simulink model "CIC_Filter_ISOP_HB"  (R2022b)
settings: Solver=FixedStepAuto  StartTime=0.0  StopTime=0.1  FixedStep=Ts/10  RelTol=1e-3
model workspace (MAT data in the model file):
  Ts = 1.953125e-06
  c = -6.248
  c6 = -5.494
settings Model: Creator=Rio  LastModifiedBy=Rio
settings DebuggingCC: ParameterPrecisionLossMsg=none

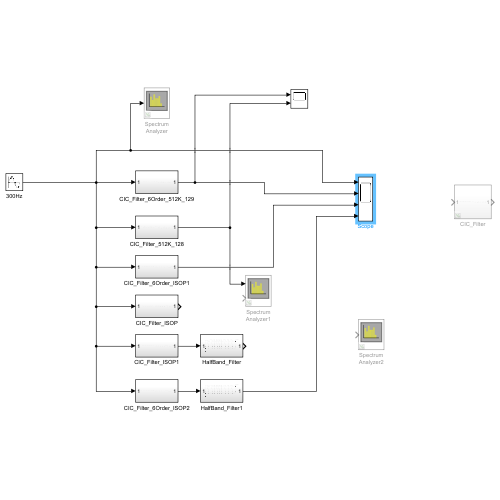
[thumbnail: Simulink's stored preview of the top-level diagram]
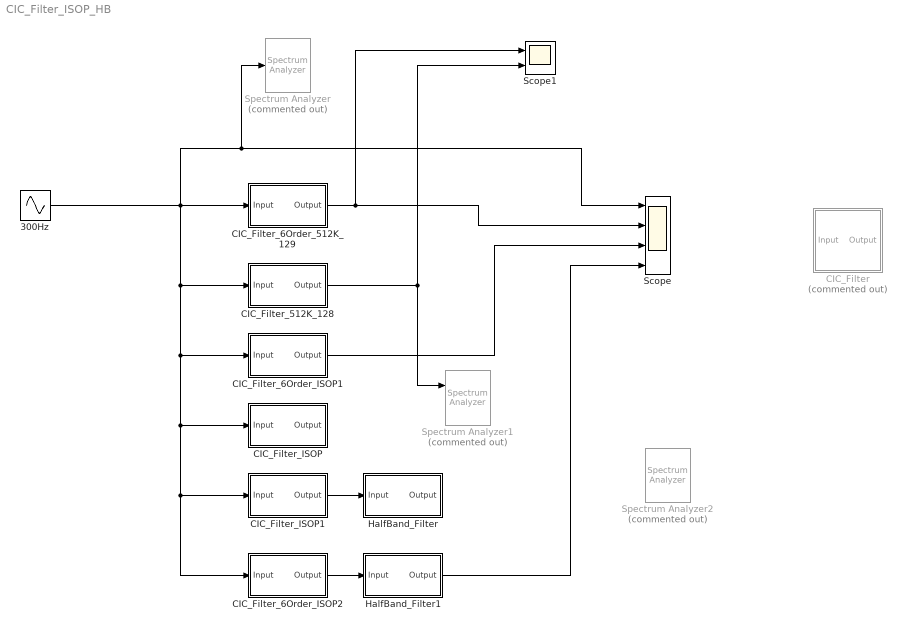
== system CIC_Filter_ISOP_HB ==
  300Hz : Sin  Frequency=2*pi*0  SampleTime=1/512000
  CIC_Filter : Subsystem  Commented=on
  CIC_Filter_512K_128 : Subsystem  Tag=FilterWizardSubSystem
      settings: ErrorFcn=dspFilterRealizedInBasicElemsAlgLoopErrFcnCallback
  CIC_Filter_6Order_512K_129 : Subsystem  Tag=FilterWizardSubSystem
      settings: ErrorFcn=dspFilterRealizedInBasicElemsAlgLoopErrFcnCallback
  CIC_Filter_6Order_ISOP1 : Subsystem  Tag=FilterWizardSubSystem
      settings: ErrorFcn=dspFilterRealizedInBasicElemsAlgLoopErrFcnCallback
  CIC_Filter_6Order_ISOP2 : Subsystem  Tag=FilterWizardSubSystem
      settings: ErrorFcn=dspFilterRealizedInBasicElemsAlgLoopErrFcnCallback
  CIC_Filter_ISOP : Subsystem  Tag=FilterWizardSubSystem
      settings: ErrorFcn=dspFilterRealizedInBasicElemsAlgLoopErrFcnCallback
  CIC_Filter_ISOP1 : Subsystem  Tag=FilterWizardSubSystem
      settings: ErrorFcn=dspFilterRealizedInBasicElemsAlgLoopErrFcnCallback
  HalfBand_Filter : Subsystem  Tag=FilterWizardSubSystem
      settings: ErrorFcn=dspFilterRealizedInBasicElemsAlgLoopErrFcnCallback
  HalfBand_Filter1 : Subsystem  Tag=FilterWizardSubSystem
      settings: ErrorFcn=dspFilterRealizedInBasicElemsAlgLoopErrFcnCallback
  Scope : Scope  NumInputPorts=4
  Scope1 : Scope  NumInputPorts=2
  Spectrum Analyzer : SpectrumAnalyzer  Commented=on
  Spectrum Analyzer1 : SpectrumAnalyzer  Commented=on  NumInputPorts=2
  Spectrum Analyzer2 : SpectrumAnalyzer  Commented=on
  wires:
  300Hz/1 -> CIC_Filter_6Order_512K_129/1(Input), CIC_Filter_6Order_ISOP1/1(Input), CIC_Filter_6Order_ISOP2/1(Input), CIC_Filter_ISOP1/1(Input), CIC_Filter_ISOP/1(Input), CIC_Filter_512K_128/1(Input), Scope/1, Spectrum Analyzer/1
  CIC_Filter_ISOP1/1(Output) -> HalfBand_Filter/1(Input)
  CIC_Filter_6Order_512K_129/1(Output) -> Scope1/1, Scope/2
  CIC_Filter_512K_128/1(Output) -> Spectrum Analyzer1/1, Scope1/2
  CIC_Filter_6Order_ISOP2/1(Output) -> HalfBand_Filter1/1(Input)
  CIC_Filter_6Order_ISOP1/1(Output) -> Scope/3
  HalfBand_Filter1/1(Output) -> Scope/4

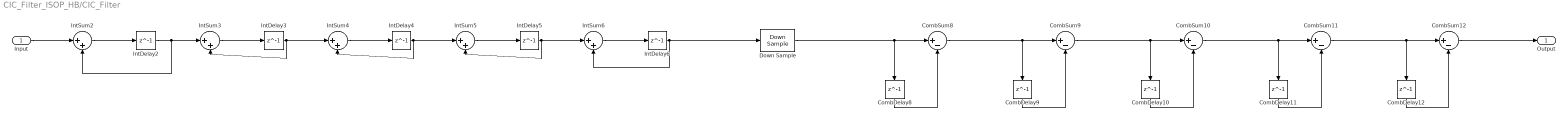
== system CIC_Filter_ISOP_HB/CIC_Filter ==
  Input : Inport
  CombDelay{8..12} (5 alike) : Delay  DelayLength=1  InitialCondition=0  SampleTime=Ts
  CombSum{8..12} (5 alike) : Sum  Inputs=|+-  AccumDataTypeStr=fixdt(1,51,15)  OutDataTypeStr=fixdt(1,51,15)
  Down Sample : DownSample  N=128  RateOptions=Allow multirate processing  AllowArbitraryFixedInput=on
  IntDelay{2..3,5..6} (4 alike) : Delay  DelayLength=1  InitialCondition=0  SampleTime=Ts
  IntDelay4 : Delay  DelayLength=1  InitialCondition=0
  IntSum{2..6} (5 alike) : Sum  Inputs=|++  AccumDataTypeStr=fixdt(1,51,15)  OutDataTypeStr=fixdt(1,51,15)
  Output : Outport
  wires:
  CombSum10/1 -> CombSum11/1, CombDelay11/1
  IntSum5/1 -> IntDelay5/1
  IntDelay4/1 -> IntSum4/2, IntSum5/1
  IntDelay6/1 -> IntSum6/2, Down Sample/1
  Down Sample/1 -> CombSum8/1, CombDelay8/1
  CombDelay12/1 -> CombSum12/2
  IntDelay5/1 -> IntSum5/2, IntSum6/1
  CombDelay8/1 -> CombSum8/2
  IntDelay3/1 -> IntSum3/2, IntSum4/1
  CombDelay11/1 -> CombSum11/2
  IntSum4/1 -> IntDelay4/1
  IntSum3/1 -> IntDelay3/1
  CombDelay10/1 -> CombSum10/2
  CombSum12/1 -> Output/1
  CombDelay9/1 -> CombSum9/2
  CombSum11/1 -> CombSum12/1, CombDelay12/1
  CombSum8/1 -> CombSum9/1, CombDelay9/1
  IntSum2/1 -> IntDelay2/1
  CombSum9/1 -> CombSum10/1, CombDelay10/1
  IntDelay2/1 -> IntSum2/2, IntSum3/1
  Input/1 -> IntSum2/1
  IntSum6/1 -> IntDelay6/1

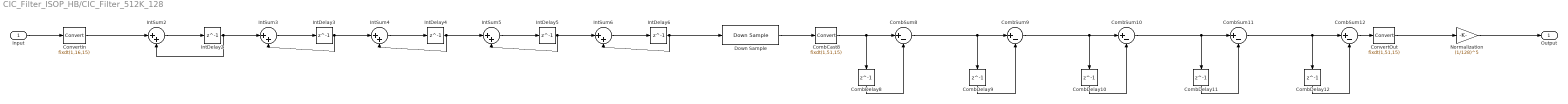
== system CIC_Filter_ISOP_HB/CIC_Filter_512K_128 ==
  Input : Inport
  CombCast8 : DataTypeConversion  OutDataTypeStr=fixdt(1,51,15)  SaturateOnIntegerOverflow=off  RndMeth=Floor
  CombDelay{8..12} (5 alike) : Delay  DelayLength=1  InitialCondition=0
  CombSum{8..12} (5 alike) : Sum  Inputs=|+-  AccumDataTypeStr=fixdt(1,51,15)  OutDataTypeStr=fixdt(1,51,15)
  ConvertIn : DataTypeConversion  OutDataTypeStr=fixdt(1,16,15)  RndMeth=Nearest
  ConvertOut : DataTypeConversion  OutDataTypeStr=fixdt(1,51,15)  SaturateOnIntegerOverflow=off  RndMeth=Floor
  Down Sample : DownSample  N=128  RateOptions=Allow multirate processing  AllowArbitraryFixedInput=on
  IntDelay{2..6} (5 alike) : Delay  DelayLength=1  InitialCondition=0
  IntSum{2..6} (5 alike) : Sum  Inputs=|++  AccumDataTypeStr=fixdt(1,51,15)  OutDataTypeStr=fixdt(1,51,15)
  Normalization : Gain  Gain=(1/128)^5
  Output : Outport
  wires:
  Input/1 -> ConvertIn/1
  IntSum2/1 -> IntDelay2/1
  IntDelay2/1 -> IntSum2/2, IntSum3/1
  IntSum3/1 -> IntDelay3/1
  IntDelay3/1 -> IntSum3/2, IntSum4/1
  IntSum4/1 -> IntDelay4/1
  IntDelay4/1 -> IntSum4/2, IntSum5/1
  IntSum5/1 -> IntDelay5/1
  IntDelay5/1 -> IntSum5/2, IntSum6/1
  IntSum6/1 -> IntDelay6/1
  IntDelay6/1 -> IntSum6/2, Down Sample/1
  Down Sample/1 -> CombCast8/1
  CombSum8/1 -> CombSum9/1, CombDelay9/1
  CombDelay8/1 -> CombSum8/2
  CombCast8/1 -> CombSum8/1, CombDelay8/1
  CombSum9/1 -> CombSum10/1, CombDelay10/1
  CombDelay9/1 -> CombSum9/2
  CombSum10/1 -> CombSum11/1, CombDelay11/1
  CombDelay10/1 -> CombSum10/2
  CombSum11/1 -> CombSum12/1, CombDelay12/1
  CombDelay11/1 -> CombSum11/2
  CombSum12/1 -> ConvertOut/1
  CombDelay12/1 -> CombSum12/2
  ConvertOut/1 -> Normalization/1
  ConvertIn/1 -> IntSum2/1
  Normalization/1 -> Output/1

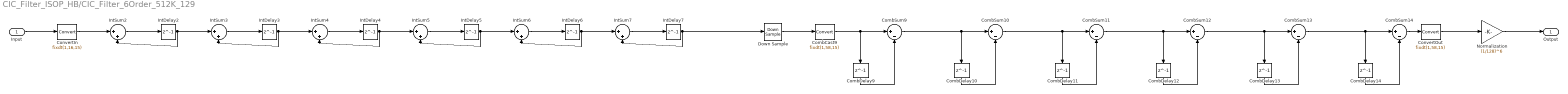
== system CIC_Filter_ISOP_HB/CIC_Filter_6Order_512K_129 ==
  Input : Inport
  CombCast9 : DataTypeConversion  OutDataTypeStr=fixdt(1,58,15)  SaturateOnIntegerOverflow=off  RndMeth=Floor
  CombDelay{9..14} (6 alike) : Delay  DelayLength=1  InitialCondition=0
  CombSum{9..14} (6 alike) : Sum  Inputs=|+-  AccumDataTypeStr=fixdt(1,58,15)  OutDataTypeStr=fixdt(1,58,15)
  ConvertIn : DataTypeConversion  OutDataTypeStr=fixdt(1,16,15)  RndMeth=Nearest
  ConvertOut : DataTypeConversion  OutDataTypeStr=fixdt(1,58,15)  SaturateOnIntegerOverflow=off  RndMeth=Floor
  Down Sample : DownSample  N=128  RateOptions=Allow multirate processing  AllowArbitraryFixedInput=on
  IntDelay{2..7} (6 alike) : Delay  DelayLength=1  InitialCondition=0
  IntSum{2..7} (6 alike) : Sum  Inputs=|++  AccumDataTypeStr=fixdt(1,58,15)  OutDataTypeStr=fixdt(1,58,15)
  Normalization : Gain  Gain=(1/128)^6
  Output : Outport
  wires:
  Input/1 -> ConvertIn/1
  ConvertIn/1 -> IntSum2/1
  IntSum2/1 -> IntDelay2/1
  IntDelay2/1 -> IntSum2/2, IntSum3/1
  IntSum3/1 -> IntDelay3/1
  IntDelay3/1 -> IntSum3/2, IntSum4/1
  IntSum4/1 -> IntDelay4/1
  IntDelay4/1 -> IntSum4/2, IntSum5/1
  IntSum5/1 -> IntDelay5/1
  IntDelay5/1 -> IntSum5/2, IntSum6/1
  IntSum6/1 -> IntDelay6/1
  IntDelay6/1 -> IntSum6/2, IntSum7/1
  IntSum7/1 -> IntDelay7/1
  IntDelay7/1 -> IntSum7/2, Down Sample/1
  Down Sample/1 -> CombCast9/1
  CombSum9/1 -> CombSum10/1, CombDelay10/1
  CombDelay9/1 -> CombSum9/2
  CombCast9/1 -> CombSum9/1, CombDelay9/1
  CombSum10/1 -> CombSum11/1, CombDelay11/1
  CombDelay10/1 -> CombSum10/2
  CombSum11/1 -> CombSum12/1, CombDelay12/1
  CombDelay11/1 -> CombSum11/2
  CombSum12/1 -> CombSum13/1, CombDelay13/1
  CombDelay12/1 -> CombSum12/2
  CombSum13/1 -> CombSum14/1, CombDelay14/1
  CombDelay13/1 -> CombSum13/2
  CombSum14/1 -> ConvertOut/1
  CombDelay14/1 -> CombSum14/2
  ConvertOut/1 -> Normalization/1
  Normalization/1 -> Output/1

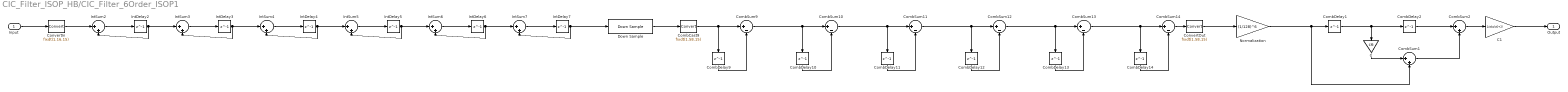
== system CIC_Filter_ISOP_HB/CIC_Filter_6Order_ISOP1 ==
  Input : Inport
  C : Gain  Gain=c6
  C1 : Gain  Gain=1/abs(c6+2)
  CombCast9 : DataTypeConversion  OutDataTypeStr=fixdt(1,58,15)  SaturateOnIntegerOverflow=off  RndMeth=Floor
  CombDelay{1..2,9..14} (8 alike) : Delay  DelayLength=1  InitialCondition=0
  CombSum1 : Sum  Inputs=|++  AccumDataTypeStr=fixdt(1,51,15)  OutDataTypeStr=fixdt(1,51,15)
  CombSum{9..14} (6 alike) : Sum  Inputs=|+-  AccumDataTypeStr=fixdt(1,58,15)  OutDataTypeStr=fixdt(1,58,15)
  CombSum2 : Sum  Inputs=|++  AccumDataTypeStr=fixdt(1,51,15)  OutDataTypeStr=fixdt(1,51,15)
  ConvertIn : DataTypeConversion  OutDataTypeStr=fixdt(1,16,15)  RndMeth=Nearest
  ConvertOut : DataTypeConversion  OutDataTypeStr=fixdt(1,58,15)  SaturateOnIntegerOverflow=off  RndMeth=Floor
  Down Sample : DownSample  N=128  RateOptions=Allow multirate processing  AllowArbitraryFixedInput=on
  IntDelay{2..7} (6 alike) : Delay  DelayLength=1  InitialCondition=0
  IntSum{2..7} (6 alike) : Sum  Inputs=|++  AccumDataTypeStr=fixdt(1,58,15)  OutDataTypeStr=fixdt(1,58,15)
  Normalization : Gain  Gain=(1/128)^6  OutDataTypeStr=Inherit: Same as input
  Output : Outport
  wires:
  ConvertOut/1 -> Normalization/1
  CombDelay14/1 -> CombSum14/2
  CombSum14/1 -> ConvertOut/1
  CombDelay13/1 -> CombSum13/2
  CombSum13/1 -> CombDelay14/1, CombSum14/1
  CombDelay12/1 -> CombSum12/2
  CombSum12/1 -> CombDelay13/1, CombSum13/1
  CombDelay11/1 -> CombSum11/2
  CombSum11/1 -> CombDelay12/1, CombSum12/1
  CombDelay10/1 -> CombSum10/2
  CombSum10/1 -> CombDelay11/1, CombSum11/1
  CombCast9/1 -> CombDelay9/1, CombSum9/1
  CombDelay9/1 -> CombSum9/2
  CombSum9/1 -> CombDelay10/1, CombSum10/1
  Down Sample/1 -> CombCast9/1
  IntDelay7/1 -> Down Sample/1, IntSum7/2
  IntSum7/1 -> IntDelay7/1
  IntDelay6/1 -> IntSum7/1, IntSum6/2
  IntSum6/1 -> IntDelay6/1
  IntDelay5/1 -> IntSum6/1, IntSum5/2
  IntSum5/1 -> IntDelay5/1
  IntDelay4/1 -> IntSum5/1, IntSum4/2
  IntSum4/1 -> IntDelay4/1
  IntDelay3/1 -> IntSum4/1, IntSum3/2
  IntSum3/1 -> IntDelay3/1
  IntDelay2/1 -> IntSum3/1, IntSum2/2
  IntSum2/1 -> IntDelay2/1
  ConvertIn/1 -> IntSum2/1
  Input/1 -> ConvertIn/1
  CombSum1/1 -> CombSum2/2
  CombDelay1/1 -> CombDelay2/1, C/1
  C1/1 -> Output/1
  C/1 -> CombSum1/1
  CombSum2/1 -> C1/1
  CombDelay2/1 -> CombSum2/1
  Normalization/1 -> CombDelay1/1, CombSum1/2

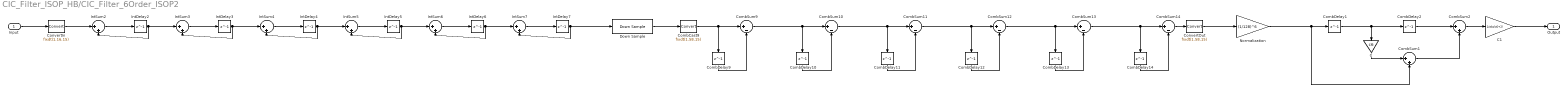
== system CIC_Filter_ISOP_HB/CIC_Filter_6Order_ISOP2 ==
  Input : Inport
  C : Gain  Gain=c6
  C1 : Gain  Gain=1/abs(c6+2)
  CombCast9 : DataTypeConversion  OutDataTypeStr=fixdt(1,58,15)  SaturateOnIntegerOverflow=off  RndMeth=Floor
  CombDelay{1..2,9..14} (8 alike) : Delay  DelayLength=1  InitialCondition=0
  CombSum1 : Sum  Inputs=|++  AccumDataTypeStr=fixdt(1,51,15)  OutDataTypeStr=fixdt(1,51,15)
  CombSum{9..14} (6 alike) : Sum  Inputs=|+-  AccumDataTypeStr=fixdt(1,58,15)  OutDataTypeStr=fixdt(1,58,15)
  CombSum2 : Sum  Inputs=|++  AccumDataTypeStr=fixdt(1,51,15)  OutDataTypeStr=fixdt(1,51,15)
  ConvertIn : DataTypeConversion  OutDataTypeStr=fixdt(1,16,15)  RndMeth=Nearest
  ConvertOut : DataTypeConversion  OutDataTypeStr=fixdt(1,58,15)  SaturateOnIntegerOverflow=off  RndMeth=Floor
  Down Sample : DownSample  N=128  RateOptions=Allow multirate processing  AllowArbitraryFixedInput=on
  IntDelay{2..7} (6 alike) : Delay  DelayLength=1  InitialCondition=0
  IntSum{2..7} (6 alike) : Sum  Inputs=|++  AccumDataTypeStr=fixdt(1,58,15)  OutDataTypeStr=fixdt(1,58,15)
  Normalization : Gain  Gain=(1/128)^6  OutDataTypeStr=Inherit: Same as input
  Output : Outport
  wires:
  Normalization/1 -> CombSum1/2, CombDelay1/1
  CombDelay2/1 -> CombSum2/1
  CombSum2/1 -> C1/1
  C/1 -> CombSum1/1
  C1/1 -> Output/1
  CombDelay1/1 -> C/1, CombDelay2/1
  CombSum1/1 -> CombSum2/2
  Input/1 -> ConvertIn/1
  ConvertIn/1 -> IntSum2/1
  IntSum2/1 -> IntDelay2/1
  IntDelay2/1 -> IntSum2/2, IntSum3/1
  IntSum3/1 -> IntDelay3/1
  IntDelay3/1 -> IntSum3/2, IntSum4/1
  IntSum4/1 -> IntDelay4/1
  IntDelay4/1 -> IntSum4/2, IntSum5/1
  IntSum5/1 -> IntDelay5/1
  IntDelay5/1 -> IntSum5/2, IntSum6/1
  IntSum6/1 -> IntDelay6/1
  IntDelay6/1 -> IntSum6/2, IntSum7/1
  IntSum7/1 -> IntDelay7/1
  IntDelay7/1 -> IntSum7/2, Down Sample/1
  Down Sample/1 -> CombCast9/1
  CombSum9/1 -> CombSum10/1, CombDelay10/1
  CombDelay9/1 -> CombSum9/2
  CombCast9/1 -> CombSum9/1, CombDelay9/1
  CombSum10/1 -> CombSum11/1, CombDelay11/1
  CombDelay10/1 -> CombSum10/2
  CombSum11/1 -> CombSum12/1, CombDelay12/1
  CombDelay11/1 -> CombSum11/2
  CombSum12/1 -> CombSum13/1, CombDelay13/1
  CombDelay12/1 -> CombSum12/2
  CombSum13/1 -> CombSum14/1, CombDelay14/1
  CombDelay13/1 -> CombSum13/2
  CombSum14/1 -> ConvertOut/1
  CombDelay14/1 -> CombSum14/2
  ConvertOut/1 -> Normalization/1

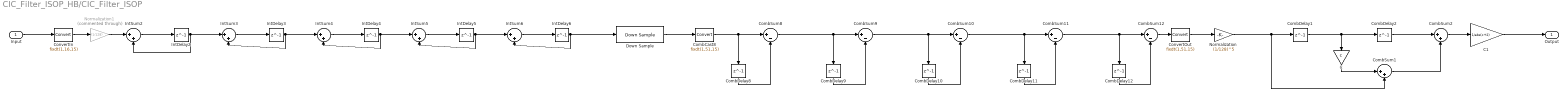
== system CIC_Filter_ISOP_HB/CIC_Filter_ISOP ==
  Input : Inport
  C : Gain  Gain=c
  C1 : Gain  Gain=1/abs(c+2)
  CombCast8 : DataTypeConversion  OutDataTypeStr=fixdt(1,51,15)  RndMeth=Floor
  CombDelay{1..2,8..12} (7 alike) : Delay  DelayLength=1  InitialCondition=0
  CombSum1 : Sum  Inputs=|++  AccumDataTypeStr=fixdt(1,51,15)  OutDataTypeStr=fixdt(1,51,15)
  CombSum{8..12} (5 alike) : Sum  Inputs=|+-  AccumDataTypeStr=fixdt(1,51,15)  OutDataTypeStr=fixdt(1,51,15)
  CombSum2 : Sum  Inputs=|++  AccumDataTypeStr=fixdt(1,51,15)  OutDataTypeStr=fixdt(1,51,15)
  ConvertIn : DataTypeConversion  OutDataTypeStr=fixdt(1,16,15)  RndMeth=Nearest
  ConvertOut : DataTypeConversion  OutDataTypeStr=fixdt(1,51,15)  RndMeth=Floor
  Down Sample : DownSample  N=128  RateOptions=Allow multirate processing  AllowArbitraryFixedInput=on
  IntDelay{2..6} (5 alike) : Delay  DelayLength=1  InitialCondition=0
  IntSum{2..6} (5 alike) : Sum  Inputs=|++  AccumDataTypeStr=fixdt(1,51,15)  OutDataTypeStr=fixdt(1,51,15)
  Normalization : Gain  Gain=(1/128)^5  OutDataTypeStr=Inherit: Same as input
  Normalization1 : Gain  Commented=through  Gain=(1/128)
  Output : Outport
  wires:
  Normalization/1 -> CombSum1/2, CombDelay1/1
  ConvertIn/1 -> Normalization1/1
  ConvertOut/1 -> Normalization/1
  CombDelay12/1 -> CombSum12/2
  CombSum12/1 -> ConvertOut/1
  CombDelay11/1 -> CombSum11/2
  CombSum11/1 -> CombDelay12/1, CombSum12/1
  CombDelay10/1 -> CombSum10/2
  CombSum10/1 -> CombDelay11/1, CombSum11/1
  CombDelay9/1 -> CombSum9/2
  CombSum9/1 -> CombDelay10/1, CombSum10/1
  CombCast8/1 -> CombDelay8/1, CombSum8/1
  CombDelay8/1 -> CombSum8/2
  CombSum8/1 -> CombDelay9/1, CombSum9/1
  Down Sample/1 -> CombCast8/1
  IntDelay6/1 -> Down Sample/1, IntSum6/2
  IntSum6/1 -> IntDelay6/1
  IntDelay5/1 -> IntSum6/1, IntSum5/2
  IntSum5/1 -> IntDelay5/1
  IntDelay4/1 -> IntSum5/1, IntSum4/2
  IntSum4/1 -> IntDelay4/1
  IntDelay3/1 -> IntSum4/1, IntSum3/2
  IntSum3/1 -> IntDelay3/1
  IntDelay2/1 -> IntSum3/1, IntSum2/2
  IntSum2/1 -> IntDelay2/1
  Input/1 -> ConvertIn/1
  CombDelay1/1 -> CombDelay2/1, C/1
  C/1 -> CombSum1/1
  CombSum1/1 -> CombSum2/2
  CombDelay2/1 -> CombSum2/1
  CombSum2/1 -> C1/1
  Normalization1/1 -> IntSum2/1
  C1/1 -> Output/1

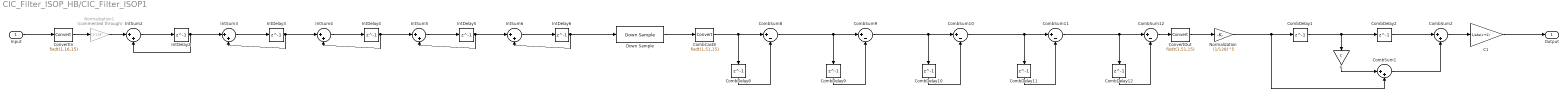
== system CIC_Filter_ISOP_HB/CIC_Filter_ISOP1 ==
  Input : Inport
  C : Gain  Gain=c
  C1 : Gain  Gain=1/abs(c+2)
  CombCast8 : DataTypeConversion  OutDataTypeStr=fixdt(1,51,15)  RndMeth=Floor
  CombDelay{1..2,8..12} (7 alike) : Delay  DelayLength=1  InitialCondition=0
  CombSum1 : Sum  Inputs=|++  AccumDataTypeStr=fixdt(1,51,15)  OutDataTypeStr=fixdt(1,51,15)
  CombSum{8..12} (5 alike) : Sum  Inputs=|+-  AccumDataTypeStr=fixdt(1,51,15)  OutDataTypeStr=fixdt(1,51,15)
  CombSum2 : Sum  Inputs=|++  AccumDataTypeStr=fixdt(1,51,15)  OutDataTypeStr=fixdt(1,51,15)
  ConvertIn : DataTypeConversion  OutDataTypeStr=fixdt(1,16,15)  RndMeth=Nearest
  ConvertOut : DataTypeConversion  OutDataTypeStr=fixdt(1,51,15)  RndMeth=Floor
  Down Sample : DownSample  N=128  RateOptions=Allow multirate processing  AllowArbitraryFixedInput=on
  IntDelay{2..6} (5 alike) : Delay  DelayLength=1  InitialCondition=0
  IntSum{2..6} (5 alike) : Sum  Inputs=|++  AccumDataTypeStr=fixdt(1,51,15)  OutDataTypeStr=fixdt(1,51,15)
  Normalization : Gain  Gain=(1/128)^5  OutDataTypeStr=Inherit: Same as input
  Normalization1 : Gain  Commented=through  Gain=(1/128)
  Output : Outport
  wires:
  C1/1 -> Output/1
  Normalization1/1 -> IntSum2/1
  CombSum2/1 -> C1/1
  CombDelay2/1 -> CombSum2/1
  CombSum1/1 -> CombSum2/2
  C/1 -> CombSum1/1
  CombDelay1/1 -> C/1, CombDelay2/1
  Input/1 -> ConvertIn/1
  IntSum2/1 -> IntDelay2/1
  IntDelay2/1 -> IntSum2/2, IntSum3/1
  IntSum3/1 -> IntDelay3/1
  IntDelay3/1 -> IntSum3/2, IntSum4/1
  IntSum4/1 -> IntDelay4/1
  IntDelay4/1 -> IntSum4/2, IntSum5/1
  IntSum5/1 -> IntDelay5/1
  IntDelay5/1 -> IntSum5/2, IntSum6/1
  IntSum6/1 -> IntDelay6/1
  IntDelay6/1 -> IntSum6/2, Down Sample/1
  Down Sample/1 -> CombCast8/1
  CombSum8/1 -> CombSum9/1, CombDelay9/1
  CombDelay8/1 -> CombSum8/2
  CombCast8/1 -> CombSum8/1, CombDelay8/1
  CombSum9/1 -> CombSum10/1, CombDelay10/1
  CombDelay9/1 -> CombSum9/2
  CombSum10/1 -> CombSum11/1, CombDelay11/1
  CombDelay10/1 -> CombSum10/2
  CombSum11/1 -> CombSum12/1, CombDelay12/1
  CombDelay11/1 -> CombSum11/2
  CombSum12/1 -> ConvertOut/1
  CombDelay12/1 -> CombSum12/2
  ConvertOut/1 -> Normalization/1
  ConvertIn/1 -> Normalization1/1
  Normalization/1 -> CombDelay1/1, CombSum1/2

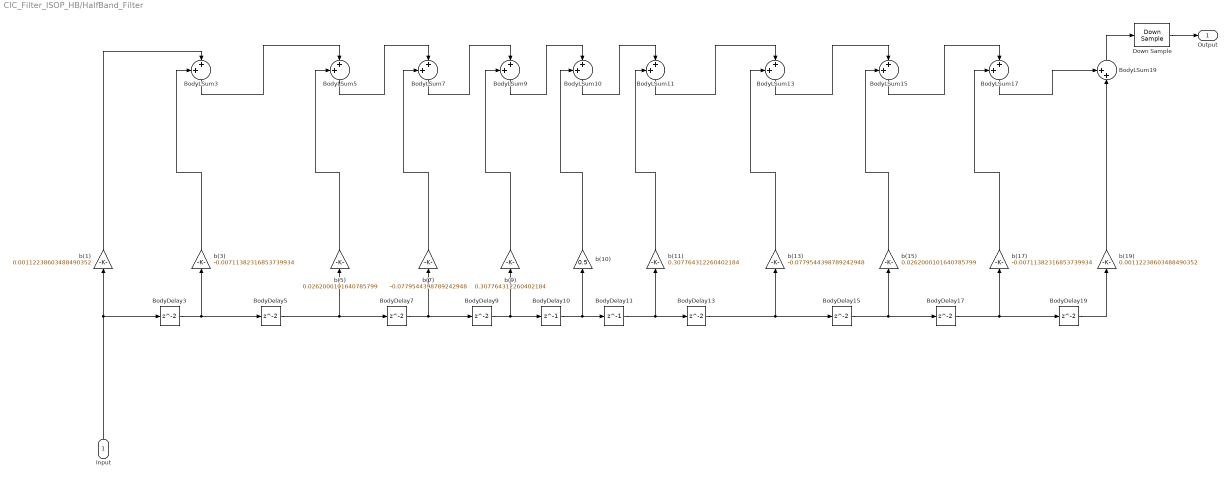
== system CIC_Filter_ISOP_HB/HalfBand_Filter ==
  Input : Inport
  BodyDelay10 : Delay  DelayLength=1  InitialCondition=0  InputProcessing=Columns as channels (frame based)
  BodyDelay11 : Delay  DelayLength=1  InitialCondition=0  InputProcessing=Columns as channels (frame based)
  BodyDelay{3,5,7,9,13,15,17,19} (8 alike) : Delay  InitialCondition=0  InputProcessing=Columns as channels (frame based)
  BodyLSum{3,5,7,9..11,13,15,17,19} (10 alike) : Sum  Inputs=++|  RndMeth=Nearest  SaturateOnIntegerOverflow=on  OutDataTypeStr=Inherit: Same as first input
  Down Sample : DownSample  RateOptions=Allow multirate processing  AllowArbitraryFixedInput=on
  b(1) : Gain  Gain=0.00112238603488490352  ParamDataTypeStr=single  RndMeth=Nearest  SaturateOnIntegerOverflow=on  OutDataTypeStr=Inherit: Same as input
  b(10) : Gain  Gain=0.5  ParamDataTypeStr=single  RndMeth=Nearest  SaturateOnIntegerOverflow=on  OutDataTypeStr=Inherit: Same as input
  b(11) : Gain  Gain=0.307764312260402184  ParamDataTypeStr=single  RndMeth=Nearest  SaturateOnIntegerOverflow=on  OutDataTypeStr=Inherit: Same as input
  b(13) : Gain  Gain=-0.0779544398789242948  ParamDataTypeStr=single  RndMeth=Nearest  SaturateOnIntegerOverflow=on  OutDataTypeStr=Inherit: Same as input
  b(15) : Gain  Gain=0.0262000101640785799  ParamDataTypeStr=single  RndMeth=Nearest  SaturateOnIntegerOverflow=on  OutDataTypeStr=Inherit: Same as input
  b(17) : Gain  Gain=-0.00711382316853739934  ParamDataTypeStr=single  RndMeth=Nearest  SaturateOnIntegerOverflow=on  OutDataTypeStr=Inherit: Same as input
  b(19) : Gain  Gain=0.00112238603488490352  ParamDataTypeStr=single  RndMeth=Nearest  SaturateOnIntegerOverflow=on  OutDataTypeStr=Inherit: Same as input
  b(3) : Gain  Gain=-0.00711382316853739934  ParamDataTypeStr=single  RndMeth=Nearest  SaturateOnIntegerOverflow=on  OutDataTypeStr=Inherit: Same as input
  b(5) : Gain  Gain=0.0262000101640785799  ParamDataTypeStr=single  RndMeth=Nearest  SaturateOnIntegerOverflow=on  OutDataTypeStr=Inherit: Same as input
  b(7) : Gain  Gain=-0.0779544398789242948  ParamDataTypeStr=single  RndMeth=Nearest  SaturateOnIntegerOverflow=on  OutDataTypeStr=Inherit: Same as input
  b(9) : Gain  Gain=0.307764312260402184  ParamDataTypeStr=single  RndMeth=Nearest  SaturateOnIntegerOverflow=on  OutDataTypeStr=Inherit: Same as input
  Output : Outport
  wires:
  Input/1 -> b(1)/1, BodyDelay3/1
  b(1)/1 -> BodyLSum3/2
  BodyDelay3/1 -> b(3)/1, BodyDelay5/1
  b(3)/1 -> BodyLSum3/1
  BodyLSum3/1 -> BodyLSum5/2
  BodyDelay5/1 -> b(5)/1, BodyDelay7/1
  b(5)/1 -> BodyLSum5/1
  BodyLSum5/1 -> BodyLSum7/2
  BodyDelay7/1 -> b(7)/1, BodyDelay9/1
  b(7)/1 -> BodyLSum7/1
  BodyLSum7/1 -> BodyLSum9/2
  BodyDelay9/1 -> b(9)/1, BodyDelay10/1
  b(9)/1 -> BodyLSum9/1
  BodyLSum9/1 -> BodyLSum10/2
  BodyDelay10/1 -> b(10)/1, BodyDelay11/1
  b(10)/1 -> BodyLSum10/1
  BodyLSum10/1 -> BodyLSum11/2
  BodyDelay11/1 -> b(11)/1, BodyDelay13/1
  b(11)/1 -> BodyLSum11/1
  BodyLSum11/1 -> BodyLSum13/2
  BodyDelay13/1 -> b(13)/1, BodyDelay15/1
  b(13)/1 -> BodyLSum13/1
  BodyLSum13/1 -> BodyLSum15/2
  BodyDelay15/1 -> b(15)/1, BodyDelay17/1
  b(15)/1 -> BodyLSum15/1
  BodyLSum15/1 -> BodyLSum17/2
  BodyDelay17/1 -> b(17)/1, BodyDelay19/1
  b(17)/1 -> BodyLSum17/1
  BodyLSum17/1 -> BodyLSum19/1
  BodyDelay19/1 -> b(19)/1
  b(19)/1 -> BodyLSum19/2
  BodyLSum19/1 -> Down Sample/1
  Down Sample/1 -> Output/1

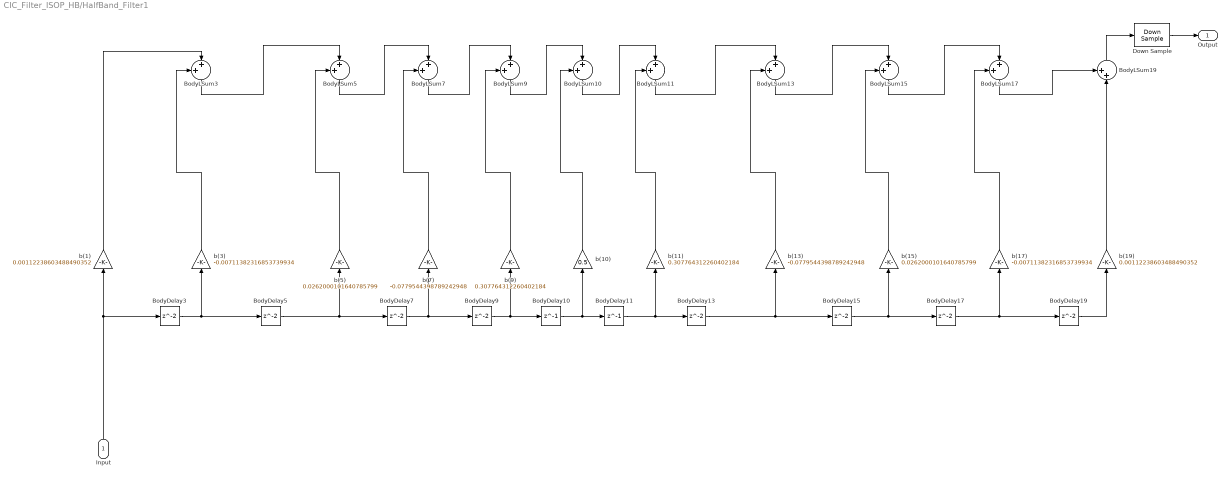
== system CIC_Filter_ISOP_HB/HalfBand_Filter1 ==
  Input : Inport
  BodyDelay10 : Delay  DelayLength=1  InitialCondition=0  InputProcessing=Columns as channels (frame based)
  BodyDelay11 : Delay  DelayLength=1  InitialCondition=0  InputProcessing=Columns as channels (frame based)
  BodyDelay{3,5,7,9,13,15,17,19} (8 alike) : Delay  InitialCondition=0  InputProcessing=Columns as channels (frame based)
  BodyLSum{3,5,7,9..11,13,15,17,19} (10 alike) : Sum  Inputs=++|  RndMeth=Nearest  SaturateOnIntegerOverflow=on  OutDataTypeStr=Inherit: Same as first input
  Down Sample : DownSample  RateOptions=Allow multirate processing  AllowArbitraryFixedInput=on
  b(1) : Gain  Gain=0.00112238603488490352  ParamDataTypeStr=single  RndMeth=Nearest  SaturateOnIntegerOverflow=on  OutDataTypeStr=Inherit: Same as input
  b(10) : Gain  Gain=0.5  ParamDataTypeStr=single  RndMeth=Nearest  SaturateOnIntegerOverflow=on  OutDataTypeStr=Inherit: Same as input
  b(11) : Gain  Gain=0.307764312260402184  ParamDataTypeStr=single  RndMeth=Nearest  SaturateOnIntegerOverflow=on  OutDataTypeStr=Inherit: Same as input
  b(13) : Gain  Gain=-0.0779544398789242948  ParamDataTypeStr=single  RndMeth=Nearest  SaturateOnIntegerOverflow=on  OutDataTypeStr=Inherit: Same as input
  b(15) : Gain  Gain=0.0262000101640785799  ParamDataTypeStr=single  RndMeth=Nearest  SaturateOnIntegerOverflow=on  OutDataTypeStr=Inherit: Same as input
  b(17) : Gain  Gain=-0.00711382316853739934  ParamDataTypeStr=single  RndMeth=Nearest  SaturateOnIntegerOverflow=on  OutDataTypeStr=Inherit: Same as input
  b(19) : Gain  Gain=0.00112238603488490352  ParamDataTypeStr=single  RndMeth=Nearest  SaturateOnIntegerOverflow=on  OutDataTypeStr=Inherit: Same as input
  b(3) : Gain  Gain=-0.00711382316853739934  ParamDataTypeStr=single  RndMeth=Nearest  SaturateOnIntegerOverflow=on  OutDataTypeStr=Inherit: Same as input
  b(5) : Gain  Gain=0.0262000101640785799  ParamDataTypeStr=single  RndMeth=Nearest  SaturateOnIntegerOverflow=on  OutDataTypeStr=Inherit: Same as input
  b(7) : Gain  Gain=-0.0779544398789242948  ParamDataTypeStr=single  RndMeth=Nearest  SaturateOnIntegerOverflow=on  OutDataTypeStr=Inherit: Same as input
  b(9) : Gain  Gain=0.307764312260402184  ParamDataTypeStr=single  RndMeth=Nearest  SaturateOnIntegerOverflow=on  OutDataTypeStr=Inherit: Same as input
  Output : Outport
  wires:
  Down Sample/1 -> Output/1
  BodyLSum19/1 -> Down Sample/1
  b(19)/1 -> BodyLSum19/2
  BodyDelay19/1 -> b(19)/1
  BodyLSum17/1 -> BodyLSum19/1
  b(17)/1 -> BodyLSum17/1
  BodyDelay17/1 -> BodyDelay19/1, b(17)/1
  BodyLSum15/1 -> BodyLSum17/2
  b(15)/1 -> BodyLSum15/1
  BodyDelay15/1 -> BodyDelay17/1, b(15)/1
  BodyLSum13/1 -> BodyLSum15/2
  b(13)/1 -> BodyLSum13/1
  BodyDelay13/1 -> BodyDelay15/1, b(13)/1
  BodyLSum11/1 -> BodyLSum13/2
  b(11)/1 -> BodyLSum11/1
  BodyDelay11/1 -> BodyDelay13/1, b(11)/1
  BodyLSum10/1 -> BodyLSum11/2
  b(10)/1 -> BodyLSum10/1
  BodyDelay10/1 -> BodyDelay11/1, b(10)/1
  BodyLSum9/1 -> BodyLSum10/2
  b(9)/1 -> BodyLSum9/1
  BodyDelay9/1 -> BodyDelay10/1, b(9)/1
  BodyLSum7/1 -> BodyLSum9/2
  b(7)/1 -> BodyLSum7/1
  BodyDelay7/1 -> BodyDelay9/1, b(7)/1
  BodyLSum5/1 -> BodyLSum7/2
  b(5)/1 -> BodyLSum5/1
  BodyDelay5/1 -> BodyDelay7/1, b(5)/1
  BodyLSum3/1 -> BodyLSum5/2
  b(3)/1 -> BodyLSum3/1
  BodyDelay3/1 -> BodyDelay5/1, b(3)/1
  b(1)/1 -> BodyLSum3/2
  Input/1 -> BodyDelay3/1, b(1)/1
